simulink model "ex5p1"  (R2016b)
settings: Solver=VariableStepAuto  StartTime=0.0  StopTime=0.3  RelTol=1e-3
InitFcn:
  | alpha = 30;
libraries: powerlib x11, simulink x6, powerlib_meascontrol x2
settings Model: Creator=user  LastModifiedBy=user

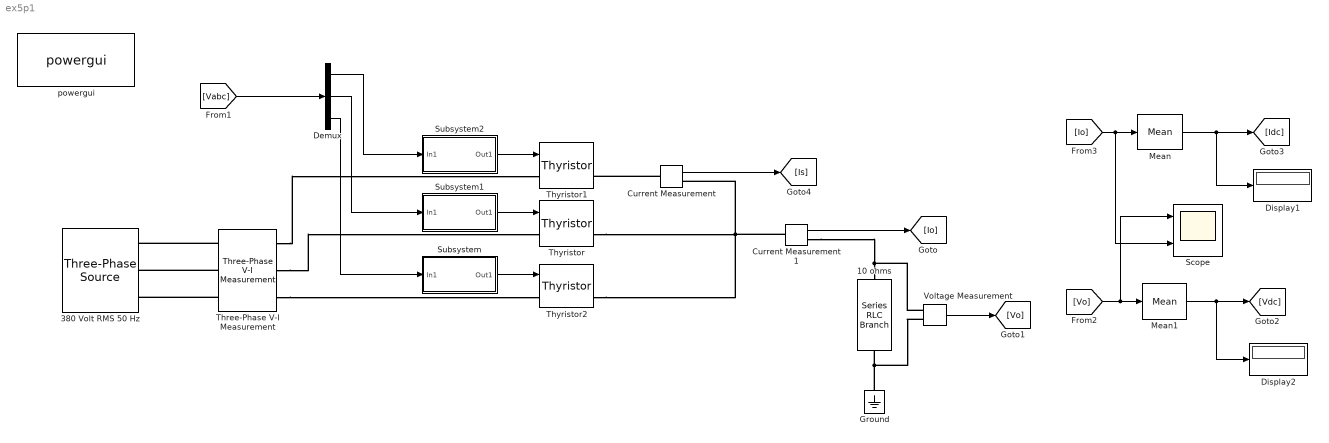
== system ex5p1 ==
  10 ohms : powerlib/Elements/Series RLC Branch  LConnTagsString=__new0  RConnTagsString=__new0  BranchType=R  Resistance=10  Inductance=0.3  SetiL0=off  InitialCurrent=0  Capacitance=1e-6  Setx0=off  InitialVoltage=0  Measurements=None
  380 Volt RMS 50 Hz : powerlib/Electrical Sources/Three-Phase Source  InternalConnection=Yg  VoltagePhases=off  Voltage=380  PhaseAngle=0  Voltage_phases=[25e3 25e3 25e3]/sqrt(3)  PhaseAngles_phases=[0 -120 +120]  Frequency=50  NonIdealSource=off  SpecifyImpedance=off  Resistance=0.8929  Inductance=16.58e-3  ShortCircuitLevel=100e6  BaseVoltage=25e3  XRratio=7  BusType=swing  Pref=10e3  Qref=0  Prefabc=[10e3, 10e3, 10e3]  Qrefabc=[0, 0, 0]  Qmin=-inf  Qmax=inf
  Current Measurement : powerlib/Measurements/Current Measurement  PhasorSimulation=off  OutputType=Complex  PSBequivalent=0
  Current Measurement1 : powerlib/Measurements/Current Measurement  PhasorSimulation=off  OutputType=Complex  PSBequivalent=0
  Demux : Demux  Outputs=3
  Display1 : Display
  Display2 : Display
  Ground : powerlib/Elements/Ground  LConnTagsString=a
  Mean : powerlib_meascontrol/Measurements/Mean  Freq=50  Vinit=0  Ts=0
  Mean1 : powerlib_meascontrol/Measurements/Mean  Freq=50  Vinit=0  Ts=0
  Scope : Scope  NumInputPorts=2
  Subsystem : Subsystem
  Subsystem1 : Subsystem
  Subsystem2 : Subsystem
  Three-Phase V-I Measurement : powerlib/Measurements/Three-Phase V-I Measurement  VoltageMeasurement=phase-to-ground  SetLabelV=on  LabelV=Vabc  Vpu=off  VpuLL=off  CurrentMeasurement=yes  SetLabelI=on  LabelI=Iabc  Ipu=off  Pbase=100e6  Vbase=500e3  OutputType=Complex  PhasorSimulation=off  PSBequivalent=0
  Thyristor : powerlib/Power Electronics/Thyristor  Ron=0.001  Lon=0  Vf=0.8  IC=0  Rs=500  Cs=250e-9  Measurements=on
  Thyristor1 : powerlib/Power Electronics/Thyristor  Ron=0.001  Lon=0  Vf=0.8  IC=0  Rs=500  Cs=250e-9  Measurements=on
  Thyristor2 : powerlib/Power Electronics/Thyristor  Ron=0.001  Lon=0  Vf=0.8  IC=0  Rs=500  Cs=250e-9  Measurements=on
  Voltage Measurement : powerlib/Measurements/Voltage Measurement  PhasorSimulation=off  OutputType=Complex  PSBequivalent=0
  powergui : powerlib/powergui  Priority=1  SimulationMode=Discrete  SolverType=Tustin/Backward Euler (TBE)  SampleTime=5e-6  frequency=60  SPID=off  DisableSnubberDevices=off  DisableRonSwitches=off  DisableVfSwitches=off  SwTol=0  DisplayEquations=off  Interpol=off  ExternalGateDelay=off  methode=off  Ts=10  FunctionMessages=off  echomessages=off  HookPort=off  EnableUseOfTLC=off  x0status=blocks  frequencyindice=50  Pbase=100e6  ErrMax=1e-4  Iterations=50  UnitsV=kV  UnitsW=MW  buscounter=0  RestoreLinks=warning  ResistiveCurrentMeasurement=off  Frange=[0:2:500]  Ylog=off  Xlog=on  ShowGrid=off  save=off  variable=ZData  structure=0  ZoomFFT=off  StartTime=0.0  cycles=1  DisplayStyle=1  fundamental=60  FreqAxis=off  MaxFrequency=1000  frequencyindicesteady=1  RmsSteady=1  display=off
  wires:
  Subsystem2/1(Out1) -> Thyristor1/1
  Subsystem1/1(Out1) -> Thyristor/1
  Subsystem/1(Out1) -> Thyristor2/1
  [Vabc] -> Demux/1
  Demux/2 -> Subsystem1/1(In1)
  Demux/1 -> Subsystem2/1(In1)
  Demux/3 -> Subsystem/1(In1)
  Voltage Measurement/1 -> [Vo]
  Current Measurement1/1 -> [Io]
  [Io] -> Scope/2, Mean/1
  Mean/1 -> Display1/1, [Idc]
  [Vo] -> Scope/1, Mean1/1
  Mean1/1 -> Display2/1, [Vdc]
  Current Measurement/1 -> [Is]
  connections:
  Three-Phase V-I Measurement/LConn1 -- 380 Volt RMS 50 Hz/RConn1
  Three-Phase V-I Measurement/LConn2 -- 380 Volt RMS 50 Hz/RConn2
  Three-Phase V-I Measurement/LConn3 -- 380 Volt RMS 50 Hz/RConn3
  Three-Phase V-I Measurement/RConn1 -- Thyristor1/LConn1
  Three-Phase V-I Measurement/RConn2 -- Thyristor/LConn1
  Three-Phase V-I Measurement/RConn3 -- Thyristor2/LConn1
  Current Measurement/LConn1 -- Thyristor1/RConn1
  Thyristor/RConn1 -- Thyristor2/RConn1 -- Current Measurement1/LConn1 -- Current Measurement/RConn1
  Current Measurement1/RConn1 -- Voltage Measurement/LConn1 -- 10 ohms/LConn1
  Ground/LConn1 -- Voltage Measurement/LConn2 -- 10 ohms/RConn1

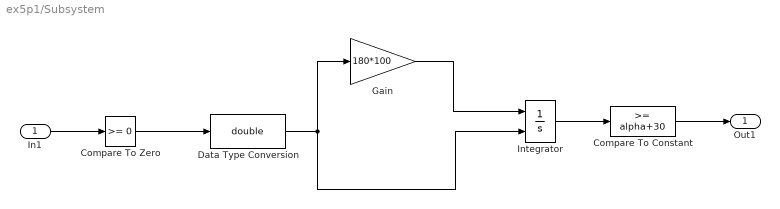
== system ex5p1/Subsystem ==
  In1 : Inport
  Compare To Constant : simulink/Logic and Bit Operations/Compare To Constant  relop=>=  const=alpha+30  OutDataTypeStr=boolean
  Compare To Zero : simulink/Logic and Bit Operations/Compare To Zero  relop=>=  OutDataTypeStr=boolean
  Data Type Conversion : DataTypeConversion  OutDataTypeStr=double
  Gain : Gain  Gain=180*100
  Integrator : Integrator  ExternalReset=falling
  Out1 : Outport
  wires:
  Data Type Conversion/1 -> Gain/1, Integrator/2
  Compare To Constant/1 -> Out1/1
  In1/1 -> Compare To Zero/1
  Integrator/1 -> Compare To Constant/1
  Compare To Zero/1 -> Data Type Conversion/1
  Gain/1 -> Integrator/1

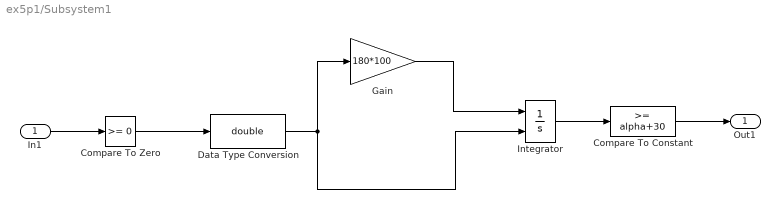
== system ex5p1/Subsystem1 ==
  In1 : Inport
  Compare To Constant : simulink/Logic and Bit Operations/Compare To Constant  relop=>=  const=alpha+30  OutDataTypeStr=boolean
  Compare To Zero : simulink/Logic and Bit Operations/Compare To Zero  relop=>=  OutDataTypeStr=boolean
  Data Type Conversion : DataTypeConversion  OutDataTypeStr=double
  Gain : Gain  Gain=180*100
  Integrator : Integrator  ExternalReset=falling
  Out1 : Outport
  wires:
  Data Type Conversion/1 -> Gain/1, Integrator/2
  Compare To Constant/1 -> Out1/1
  In1/1 -> Compare To Zero/1
  Integrator/1 -> Compare To Constant/1
  Compare To Zero/1 -> Data Type Conversion/1
  Gain/1 -> Integrator/1

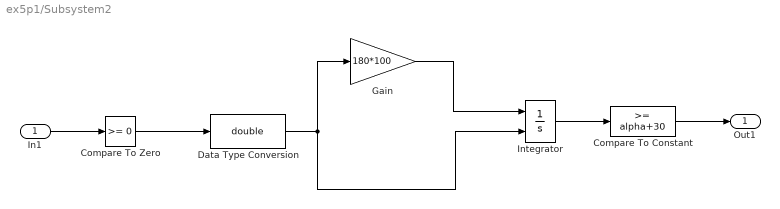
== system ex5p1/Subsystem2 ==
  In1 : Inport
  Compare To Constant : simulink/Logic and Bit Operations/Compare To Constant  relop=>=  const=alpha+30  OutDataTypeStr=boolean
  Compare To Zero : simulink/Logic and Bit Operations/Compare To Zero  relop=>=  OutDataTypeStr=boolean
  Data Type Conversion : DataTypeConversion  OutDataTypeStr=double
  Gain : Gain  Gain=180*100
  Integrator : Integrator  ExternalReset=falling
  Out1 : Outport
  wires:
  Data Type Conversion/1 -> Gain/1, Integrator/2
  Compare To Constant/1 -> Out1/1
  In1/1 -> Compare To Zero/1
  Integrator/1 -> Compare To Constant/1
  Compare To Zero/1 -> Data Type Conversion/1
  Gain/1 -> Integrator/1
